simulink model "model_jedna_zmienna"  (Simulink 10.2)
settings: Solver=VariableStepAuto  StartTime=0.0  StopTime=500000  MaxStep=0.01  RelTol=1e-3
values from neighbouring files (symbols this model uses):
  cw = 4200    [bachelor.m]
  H0 = 1    [bachelor.m]
  k = 160    [bachelor.m]
  rho = 1000    [bachelor.m]
  T0 = 20    [bachelor.m]
  Tin0 = 70    [bachelor.m]
  Vflow0 = 0.005    [bachelor.m]
  Vpl = 1.02    [bachelor.m]
settings Model: Creator=jmach  LastModifiedBy=jmach
settings DataIOCC: SaveFormat=Dataset  SignalLoggingSaveFormat=Dataset  ReturnWorkspaceOutputs=on
settings OptimizationCC: LifeSpan=auto
settings DebuggingCC: UnderspecifiedInitializationDetection=Simplified  MergeDetectMultiDrivingBlocksExec=error  FcnCallInpInsideContextMsg=error  SFUnexpectedBacktrackingDiag=error  SFNoUnconditionalDefaultTransitionDiag=error  SFExecutionAtInitializationDiag=warning  ArithmeticOperatorsInVariantConditions=error
settings HardwareCC: ProdBitPerPointer=64  ProdBitPerSizeT=64  ProdBitPerPtrDiffT=64  ProdLargestAtomicFloat=Float  ProdIntDivRoundTo=Zero  ProdEndianess=LittleEndian  ProdWordSize=64  ProdHWDeviceType=Intel->x86-64 (Windows64)
settings ModelReferenceCC: PropagateSignalLabelsOutOfModel=on
settings SFSimCC: SimUseLocalCustomCode=on  CustomCodeUndefinedFunction=FilterOut
settings RTWCC: RTWUseLocalCustomCode=on
settings CodeAppCC: StateflowObjectComments=off
settings GRTTargetCC: TargetLangStandard=C99 (ISO)  CombineOutputUpdateFcns=on  GRTInterface=off
settings ConfigComp: CovMetricSettings=dwe  CovSaveCumulativeToWorkspaceVar=off  CovSaveSingleToWorkspaceVar=off  CovExternalEMLEnable=on

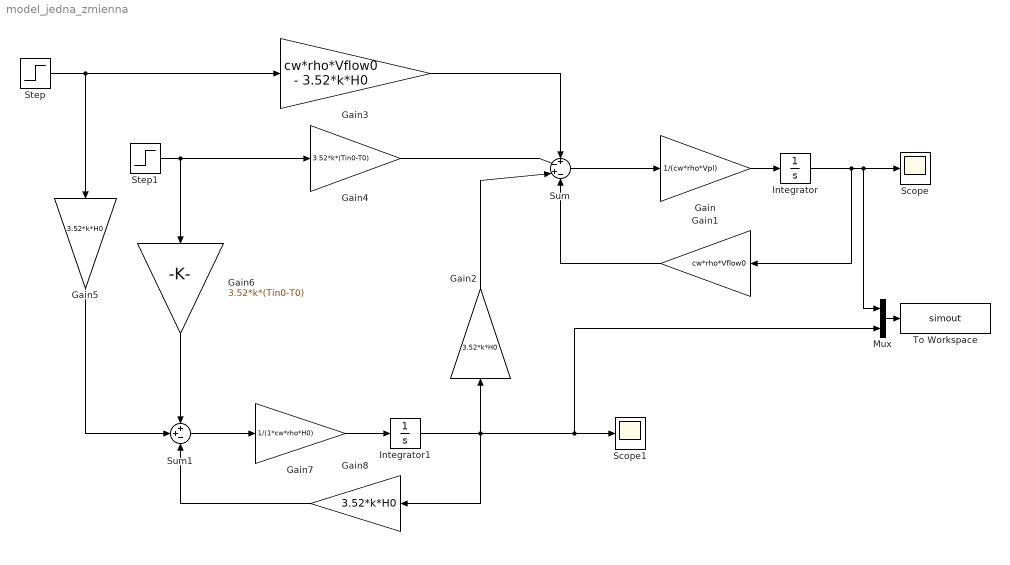
== system model_jedna_zmienna ==
  Gain : Gain  Gain=1/(cw*rho*Vpl)
  Gain1 : Gain  Gain=cw*rho*Vflow0
  Gain2 : Gain  Gain=3.52*k*H0
  Gain3 : Gain  Gain=cw*rho*Vflow0 - 3.52*k*H0
  Gain4 : Gain  Gain=3.52*k*(Tin0-T0)
  Gain5 : Gain  Gain=3.52*k*H0
  Gain6 : Gain  Gain=3.52*k*(Tin0-T0)
  Gain7 : Gain  Gain=1/(1*cw*rho*H0)
  Gain8 : Gain  Gain=3.52*k*H0
  Integrator : Integrator
  Integrator1 : Integrator
  Mux : Mux  Inputs=2
  Scope : Scope
  Scope1 : Scope
  Step : Step  Time=0  After=70  SampleTime=0
  Step1 : Step  Time=0  SampleTime=0
  Sum : Sum  Inputs=+-+-
  Sum1 : Sum  Inputs=++-
  To Workspace : ToWorkspace  VariableName=simout  SampleTime=-1
  wires:
  Sum/1 -> Gain/1
  Gain/1 -> Integrator/1
  Integrator/1 -> Gain1/1, Mux/1, Scope/1
  Gain1/1 -> Sum/4
  Gain3/1 -> Sum/1
  Gain4/1 -> Sum/2
  Gain2/1 -> Sum/3
  Gain7/1 -> Integrator1/1
  Integrator1/1 -> Mux/2, Scope1/1, Gain2/1, Gain8/1
  Sum1/1 -> Gain7/1
  Gain8/1 -> Sum1/3
  Gain6/1 -> Sum1/1
  Gain5/1 -> Sum1/2
  Mux/1 -> To Workspace/1
  Step1/1 -> Gain4/1, Gain6/1
  Step/1 -> Gain5/1, Gain3/1
